simulink model "tutorial19_robust"  (R2025a)
settings: Solver=VariableStepAuto  StartTime=0.0  StopTime=10.0  RelTol=1e-3
settings Model: Creator=xing2  LastModifiedBy=xing2

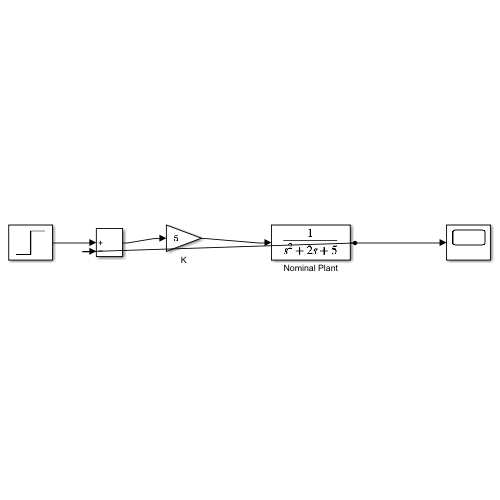
[thumbnail: Simulink's stored preview of the top-level diagram]
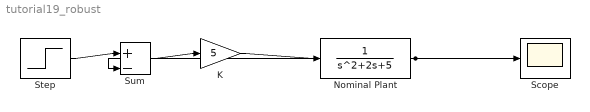
== system tutorial19_robust ==
  K : Gain  Gain=5
  Nominal Plant : TransferFcn  Denominator=[1 2 5]
  Scope : Scope
  Step : Step  Time=0.5  SampleTime=0
  Sum : Sum  Inputs=|+-
  wires:
  Step/1 -> Sum/1
  Sum/1 -> K/1
  K/1 -> Nominal Plant/1
  Nominal Plant/1 -> Scope/1, Sum/2
